simulink model "hop_mf"  (R2020b)
settings: Solver=ode45  StartTime=0.0  StopTime=150  RelTol=1e-3
libraries: simulink x2
settings Model: Creator=Stefano  LastModifiedBy=Stefano

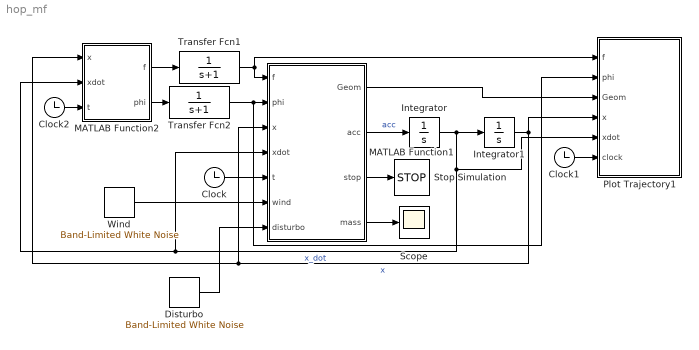
== system hop_mf ==
  Clock : Clock
  Clock1 : Clock
  Clock2 : Clock
  Disturbo : simulink/Sources/Band-Limited White Noise  Cov=[0.000001]  Ts=0.1  seed=[23341]
  Integrator : Integrator  InitialCondition=[0 0 0]
  Integrator1 : Integrator  InitialCondition=[0 20 0]
  MATLAB Function1 : MATLAB Function  TreatAsAtomicUnit=on  SystemSampleTime=0.01
  MATLAB Function2 : MATLAB Function  TreatAsAtomicUnit=on
  Plot Trajectory1 : MATLAB Function  TreatAsAtomicUnit=on  SystemSampleTime=0.1
  Scope : Scope
  Stop Simulation : Stop
  Transfer Fcn1 : TransferFcn  Denominator=[1 1]
  Transfer Fcn2 : TransferFcn  Denominator=[1 1]
  Wind : simulink/Sources/Band-Limited White Noise  Cov=[0.000000001]  Ts=0.1  seed=[23341]
  wires:
  MATLAB Function1/2(acc) -> Integrator/1  "acc"
  Integrator/1 -> Plot Trajectory1/5(xdot), MATLAB Function2/2(xdot), MATLAB Function1/4(xdot), Integrator1/1  "x_dot"
  Integrator1/1 -> MATLAB Function1/3(x), MATLAB Function2/1(x), Plot Trajectory1/4(x)  "x"
  MATLAB Function1/3(stop) -> Stop Simulation/1
  MATLAB Function1/4(mass) -> Scope/1
  Clock/1 -> MATLAB Function1/5(t)
  Clock1/1 -> Plot Trajectory1/6(clock)
  MATLAB Function1/1(Geom) -> Plot Trajectory1/3(Geom)
  Clock2/1 -> MATLAB Function2/3(t)
  Transfer Fcn1/1 -> Plot Trajectory1/1(f), MATLAB Function1/1(f)
  MATLAB Function2/1(f) -> Transfer Fcn1/1
  MATLAB Function2/2(phi) -> Transfer Fcn2/1
  Transfer Fcn2/1 -> Plot Trajectory1/2(phi), MATLAB Function1/2(phi)
  Wind/1 -> MATLAB Function1/6(wind)
  Disturbo/1 -> MATLAB Function1/7(disturbo)

== matlab function hop_mf/MATLAB Function1 ==
  data: Geom output; f input; acc output; phi input; x input; xdot input; stop output; t input; wind input; disturbo input; mass output
function [Geom,acc,stop,mass] = accelerazioni(f,phi,x,xdot,t,wind,disturbo)

% y: spostamento laterale x(1)
% z:   quota x(2)
% theta: angolo razzo x(3)
% phi: angolo di controllo dell'ugello
% f: spinta del razzo

persistent mass_consumption;

%-------------------------------------
% Inizializzazione variabili di uscita
Geom=[0 0 0];
stop=0;
acc=[0 0 0];
mass=0;

%-------------------------------------
% Parametri
M=45000;  % peso in Kg 
Dia=9; % diametro 
Alt=50; % altezza 
I=1/12*M*(Dia^2+Alt^2); % inerzia in Kg*m^2
L=20;    % distanza baricentro-ugello
g=9.8;  % accelerazione di gravitÃ 
D=M*g/100; % attrito necessario a cadere al massimo a 350 Km/h
Specific_Impulse=334; % Impulso specifico
Flow_Rate=931.2; % sea level
Fmax=(Flow_Rate*Specific_Impulse)*3; % 3 raptors

%-------------------------------------
% Saturazione della spinta
if f>Fmax
    f=Fmax;
end

%-------------------------------------
% Consumo della massa
if isempty(mass_consumption)
   mass_consumption=0; 
else
   mass_consumption=mass_consumption+0.01*f/(Specific_Impulse*3);
end
mass=M-mass_consumption;

%-------------------------------------
% Calcolo Accelerazioni
acc(1)= -f*sin(x(3)+phi)/mass+wind; 
acc(2)= -g + f/mass*cos(x(3) + phi) - D/mass*xdot(2);      
acc(3)= -L/I*sin(phi)*f+disturbo;


%-------------------------------------
% Stop alla simulazione
if x(2)<=L && t>10
     stop=1;
end

%-------------------------------------
% Sulla piattaforma di lancio/atterraggio non può andare indietro
if x(2)<L && acc(2)<0
     acc(2)=0;
end

%-------------------------------------
% Trasferimento della geometria
Geom(1)=L;
Geom(2)=Alt;
Geom(3)=Dia;

== matlab function hop_mf/Plot Trajectory1 ==
  settings: updateMethod=DISCRETE
  data: f input; phi input; Geom input; x input; xdot input; clock input
function PlotRocket(f,phi,Geom,x,xdot,clock)

eml.extrinsic('findobj','get','set','figure','clf',...
              'hold','delete','plot','axis','grid',...
              'hggroup','quiver','drawnow','num2str');
          
persistent chain;
persistent thrust;
persistent ground;
persistent deleted_fig;

%-------------------------------------
% Recupero la Geometria
L=Geom(1);
Alt=Geom(2);
Dia=Geom(3);

%-------------------------------------
% posizione del propulsore
pex=x(1)+L*sin(x(3));
pey=x(2)-L*cos(x(3));

%-------------------------------------
% Vettore di propulsione
vex=f*sin(x(3)+phi)/2000;
vey=-f*cos(x(3)+phi)/2000;

%-------------------------------------
% Gestisco la figura di output
if isempty(deleted_fig)
    deleted_fig=1;
    % La prima volta cancello la figura
    foundFig=findobj('Tag','trajScope');
    if ~isempty(foundFig)
        cla(foundFig)
    end      
else
    foundFig=findobj('Tag','trajScope');
end


%-------------------------------------
if isempty(foundFig)
    fig=figure('Color','white');
    clf(fig);
    set(fig,'Name','Trajectory');
    set(fig,'DoubleBuffer','on','Tag','trajScope');
    set(fig,'Renderer','painters');
    hold('on');
    hax=get(fig,'CurrentAxes');
    set(hax,'DrawMode','fast','Box','off');    
    

    chain=hggroup;
    thrust=quiver(hax,pex,pey,vex,vey,'Color','green','LineWidth',2);
    ground=plot([-30 30],[0 0],'c','LineWidth',3);
    grid('on');
    
else
    
    hax=get(foundFig,'CurrentAxes');

end


if ~isempty(chain)
    delete(chain);
    delete(thrust);
end



% draw the center of mass
chain=hggroup;
h1=plot(hax,x(1),x(2),'r*','LineWidth',3);


width = Dia; % whatever
height = (Alt-L)*2/3; % whatever...
xLeft = - width/2;
xRigth = width/2;
yBottom = - L;
yTop = height;
xPoint=0;
yPoint=height*3/2;

Vertex=[xLeft yTop  1
        xPoint yPoint 1
        xRigth yTop  1
        xRigth yBottom 1
        xLeft  yBottom 1
        xLeft yTop  1];
    
Rot=[cos(-x(3))  sin(-x(3)) x(1)
     -sin(-x(3)) cos(-x(3)) x(2)
      0         0        1];
      
Vertex=(Rot*Vertex')';

h2=line(Vertex(:,1),Vertex(:,2));


%h2=rectangle('Position', [xLeft, yBottom, width, height], 'EdgeColor', 'b', 'FaceColor', 'r', 'LineWidth', 4);

set(h1,'Parent',chain);
set(h2,'Parent',chain);



% draw the thrust

thrust=quiver(hax,pex,pey,vex,vey,'Color','green','LineWidth',2);


% draw the ground
if x(2)<100
    if isempty(ground)
        ground=plot([-30 30],[0 0],'c','LineWidth',3);
    end
end


xlabel(num2str(xdot(2)))
%axis([-2 42 0 102])
axis equal
drawnow;

== matlab function hop_mf/MATLAB Function2 ==
  data: x input; f output; xdot input; t input; phi output
function [f,phi] = fcn(x,xdot,t)
y=x(1);
z=x(2);
theta=x(3);

% Proporzionale derivativo
Kp=4;
Kd=10;
phi=Kp*theta+Kd*xdot(3);


if t<20
    f=900000;
else
   v_des=-x(2)/20;
   f=200000*(v_des-xdot(2)); 
end


if f<0
    f=0;
end
